simulink model "DCMotorModellingWithLoad"  (R2020b)
settings: Solver=VariableStepAuto  StartTime=0.0  StopTime=10.0  RelTol=1e-3
undefined symbols (not defined in the file): B, J, K, La, Ra
libraries: simulink_extras x2
settings Model: Creator=Bhargav  LastModifiedBy=Bhargav

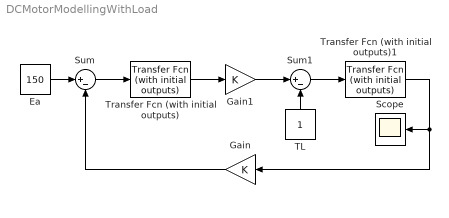
== system DCMotorModellingWithLoad ==
  Ea : Constant  Value=150
  Gain : Gain  Gain=K
  Gain1 : Gain  Gain=K
  Scope : Scope
  Sum : Sum  Inputs=|+-
  Sum1 : Sum  Inputs=|+-
  TL : Constant
  Transfer Fcn (with initial outputs) : simulink_extras/Additional Linear/Transfer Fcn (with initial outputs)  N=[1]  D=[La Ra]  Y0=0  U0=0
  Transfer Fcn (with initial outputs)1 : simulink_extras/Additional Linear/Transfer Fcn (with initial outputs)  N=[1]  D=[J B]  Y0=0  U0=0
  wires:
  Ea/1 -> Sum/1
  Sum/1 -> Transfer Fcn (with initial outputs)/1
  Transfer Fcn (with initial outputs)/1 -> Gain1/1
  Gain1/1 -> Sum1/1
  Sum1/1 -> Transfer Fcn (with initial outputs)1/1
  TL/1 -> Sum1/2
  Gain/1 -> Sum/2
  Transfer Fcn (with initial outputs)1/1 -> Scope/1, Gain/1
